simulink model "TIApplication"  (R2023b)
settings: Solver=FixedStepAuto  StartTime=0.0  StopTime=Inf  RelTol=1e-3  EnableMultiTasking=on
undefined symbols (not defined in the file): CountPerVolt, CurrentControl_I, CurrentControl_P, CurrentSensor_Bias, CurrentSensor_Gain, Down, FastSim_ElecTs, GPTRIP1SEL, GPTRIP2SEL, inverterBusVoltage, InverterCurrent_Max, InverterDCLink_Voltage, K, Ld, Lq, M, p, psim, pwmCounterMax, PWMMod_Period, PWMPercentAtZeroVolt, PWMPercentPerVolt, SpeedControl_I, SpeedControl_P, TI_ADCMax, TI_ADCMin, TI_ADCResolution, Tmax, TransducerVoltAtZeroAmpere, TransduceVoltPerAmpere, Ts, TZ1, TZ2, Up, ZeroVoltCount
libraries: mcbcontrolslib x9, c2802xlib x7, simulink x3, mcbpositiondecoderlib x3, slpidlib x3, idelinklib_common x2, c280xlib x2, mcbhdlpositiondecoderlib x2, eePmsmCurrentController x1, eeTransforms x1, eePwmGeneratorTwoLevel x1, eeLuenbergerObserver x1
(part 2 of 2)

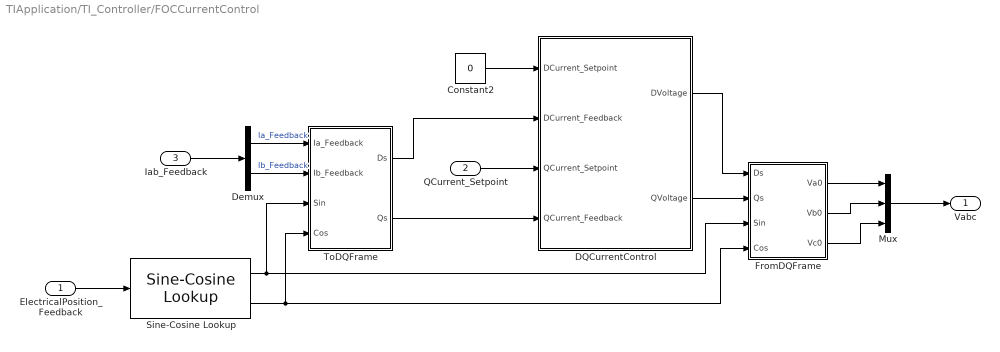
== system TIApplication/TI_Controller/FOCCurrentControl ==
  ElectricalPosition_Feedback : Inport
  QCurrent_Setpoint : Inport  Port=2
  Iab_Feedback : Inport  Port=3
  Constant2 : Constant  Value=0  OutDataTypeStr=Inherit: Inherit via back propagation  SampleTime=-1
  DQCurrentControl : Subsystem
  Demux : Demux  Outputs=2
  FromDQFrame : Subsystem
  Mux : Mux  Inputs=3
  Sine-Cosine Lookup : mcbcontrolslib/Sine-Cosine Lookup  AngleInput=Radians  N_points=1024
      settings: LibrarySourceBlock=mcblib/Controls/Math Transforms/Sine-Cosine Lookup
  ToDQFrame : Subsystem
  Vabc : Outport
  wires:
  Sine-Cosine Lookup/2 -> FromDQFrame/4(Cos), ToDQFrame/4(Cos)
  QCurrent_Setpoint/1 -> DQCurrentControl/3(QCurrent_Setpoint)
  Iab_Feedback/1 -> Demux/1
  Sine-Cosine Lookup/1 -> FromDQFrame/3(Sin), ToDQFrame/3(Sin)
  Constant2/1 -> DQCurrentControl/1(DCurrent_Setpoint)
  Mux/1 -> Vabc/1
  ElectricalPosition_Feedback/1 -> Sine-Cosine Lookup/1
  Demux/1 -> ToDQFrame/1(Ia_Feedback)  "Ia_Feedback"
  Demux/2 -> ToDQFrame/2(Ib_Feedback)  "Ib_Feedback"
  ToDQFrame/1(Ds) -> DQCurrentControl/2(DCurrent_Feedback)
  ToDQFrame/2(Qs) -> DQCurrentControl/4(QCurrent_Feedback)
  DQCurrentControl/1(DVoltage) -> FromDQFrame/1(Ds)
  DQCurrentControl/2(QVoltage) -> FromDQFrame/2(Qs)
  FromDQFrame/1(Va0) -> Mux/1
  FromDQFrame/2(Vb0) -> Mux/2
  FromDQFrame/3(Vc0) -> Mux/3

== system TIApplication/TI_Controller/PUToPWMPercent ==
  Vabc : Inport
  Add : Sum
  Constant : Constant  Value=PWMPercentPerVolt  OutDataTypeStr=Inherit: Inherit via back propagation  SampleTime=-1
  Constant2 : Constant  Value=PWMPercentAtZeroVolt  OutDataTypeStr=Inherit: Inherit via back propagation  SampleTime=-1
  Data Type Conversion : DataTypeConversion  OutDataTypeStr=uint16  SaturateOnIntegerOverflow=off  RndMeth=Floor
  Product : Product  OutDataTypeStr=Inherit: Inherit via back propagation
  Saturation : Saturate  UpperLimit=100  LowerLimit=0
  DutyCyclePercent : Outport
  wires:
  Vabc/1 -> Product/1
  Add/1 -> Saturation/1
  Constant/1 -> Product/2
  Product/1 -> Add/1
  Constant2/1 -> Add/2
  Saturation/1 -> Data Type Conversion/1
  Data Type Conversion/1 -> DutyCyclePercent/1

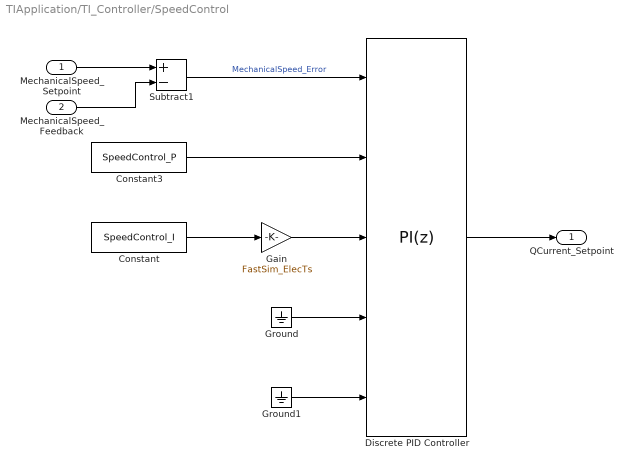
== system TIApplication/TI_Controller/SpeedControl ==
  MechanicalSpeed_Setpoint : Inport
  MechanicalSpeed_Feedback : Inport  Port=2
  Constant : Constant  Value=SpeedControl_I  OutDataTypeStr=Inherit: Inherit via back propagation  SampleTime=-1
  Constant3 : Constant  Value=SpeedControl_P  OutDataTypeStr=Inherit: Inherit via back propagation  SampleTime=-1
  Discrete PID Controller : slpidlib/PID Controller  Controller=PI  Form=Parallel  TimeDomain=Discrete-time  UseExternalTs=off  SampleTime=-1  IntegratorMethod=Forward Euler  FilterMethod=Forward Euler  ControllerParametersSource=external  P=1  I=1  UseKiTs=on  D=0  N=100  UseFilter=on  TunerSelectOption=Transfer Function Based (PID Tuner App)  InitialConditionSource=external  InitialConditionForIntegrator=0  InitialConditionForFilter=0  DifferentiatorICPrevScaledInput=0  ExternalReset=level  TrackingMode=off  Kt=1  LimitOutput=on  SatLimitsSource=internal  UpperSaturationLimit=InverterCurrent_Max  LowerSaturationLimit=-InverterCurrent_Max  LinearizeAsGain=on  AntiWindupMode=none  Kb=1  LimitIntegrator=off  UpperIntegratorSaturationLimit=inf  LowerIntegratorSaturationLimit=-inf  RndMeth=Simplest  POutMin=[]  POutMax=[]  IOutMin=[]  IOutMax=[]  DOutMin=[]  DOutMax=[]  NOutMin=[]  NOutMax=[]  SumOutMin=[]  SumOutMax=[]  SaturationOutMin=[]  SaturationOutMax=[]  PParamMin=[]  PParamMax=[]  IParamMin=[]  IParamMax=[]  DParamMin=[]  DParamMax=[]  NParamMin=[]  NParamMax=[]  KbParamMin=[]  KbParamMax=[]  KtParamMin=[]  KtParamMax=[]  KbOutMin=[]  KbOutMax=[]  KtOutMin=[]  KtOutMax=[]  IntegratorOutMin=[]  IntegratorOutMax=[]  FilterOutMin=[]  FilterOutMax=[]  SumI1OutMin=[]  SumI1OutMax=[]  SumI2OutMin=[]  SumI2OutMax=[]  SumI3OutMin=[]  SumI3OutMax=[]  SumI4OutMin=[]  SumI4OutMax=[]  SumDOutMin=[]  SumDOutMax=[]  DifferentiatorOutMin=[]  DifferentiatorOutMax=[]  FilterDiffOutCoefMin=[]  FilterDiffOutCoefMax=[]  ReciprocalOutMin=[]  ReciprocalOutMax=[]  SumDenOutMin=[]  SumDenOutMax=[]  SumNumOutMin=[]  SumNumOutMax=[]  DivideOutMin=[]  DivideOutMax=[]  UdiffTsProdOutMin=[]  UdiffTsProdOutMax=[]  NTsProdOutMin=[]  NTsProdOutMax=[]  UintegralTsProdOutMin=[]  UintegralTsProdOutMax=[]  UngainTsProdOutMin=[]  UngainTsProdOutMax=[]  ClampingZeroOutDataTypeStr=Inherit: Inherit via back propagation  ClampingZeroOutMin=[]  ClampingZeroOutMax=[]  FilterDenConstantOutDataTypeStr=Inherit: Inherit via back propagation  FilterDenConstantOutMin=[]  FilterDenConstantOutMax=[]  PCopyOutDataTypeStr=Inherit: Inherit via back propagation  PCopyOutMin=[]  PCopyOutMax=[]  NCopyOutDataTypeStr=Inherit: Inherit via back propagation  NCopyOutMin=[]  NCopyOutMax=[]  IntegratorContinuousStateAttributes=''  IntegratorStateMustResolveToSignalObject=off  IntegratorRTWStateStorageClass=Auto  FilterContinuousStateAttributes=''  FilterStateMustResolveToSignalObject=off  FilterRTWStateStorageClass=Auto  ParallelPVariant=ExternalParameters  IdealPVariant=Disabled  IVariant=ExternalParameters  DVariant=Disabled  IntegratorVariant=Discrete  SatVariant=Enabled  AWVariant=Passthrough  PCopyVariant=Disabled  TRVariant=Disabled  FdbkBlocksVariant=Forward  IdealPFdbkVariant=Disabled  SatFdbkVariant=Disabled  DerivativeFilterVariant=Disabled  NVariant=Disabled  NCopyVariant=Disabled_SignalSpec  FilterICVariant=Disabled  IntegratorICVariant=ExternalICs  ExternalResetVariant=ExternalReset  TRSumVariant=Passthrough  SumFdbkVariant=Disabled  SumVariant=Sum_PI  TsampFilterVariant=InternalTs  TsampNgainVariant=Passthrough  TsampIntegralVariant=Disabled_SignalSpec  ExternalSaturationOutDataTypeStr=Inherit: Same as second input
      settings: LibrarySourceBlock=simulink/Discrete/Discrete PID Controller
  Gain : Gain  Gain=FastSim_ElecTs
  Ground : Ground
  Ground1 : Ground
  Subtract1 : Sum  Inputs=+-
  QCurrent_Setpoint : Outport
  wires:
  Constant/1 -> Gain/1
  MechanicalSpeed_Feedback/1 -> Subtract1/2
  Ground/1 -> Discrete PID Controller/4
  Subtract1/1 -> Discrete PID Controller/1  "MechanicalSpeed_Error"
  Constant3/1 -> Discrete PID Controller/2
  Gain/1 -> Discrete PID Controller/3
  Discrete PID Controller/1 -> QCurrent_Setpoint/1
  MechanicalSpeed_Setpoint/1 -> Subtract1/1
  Ground1/1 -> Discrete PID Controller/5

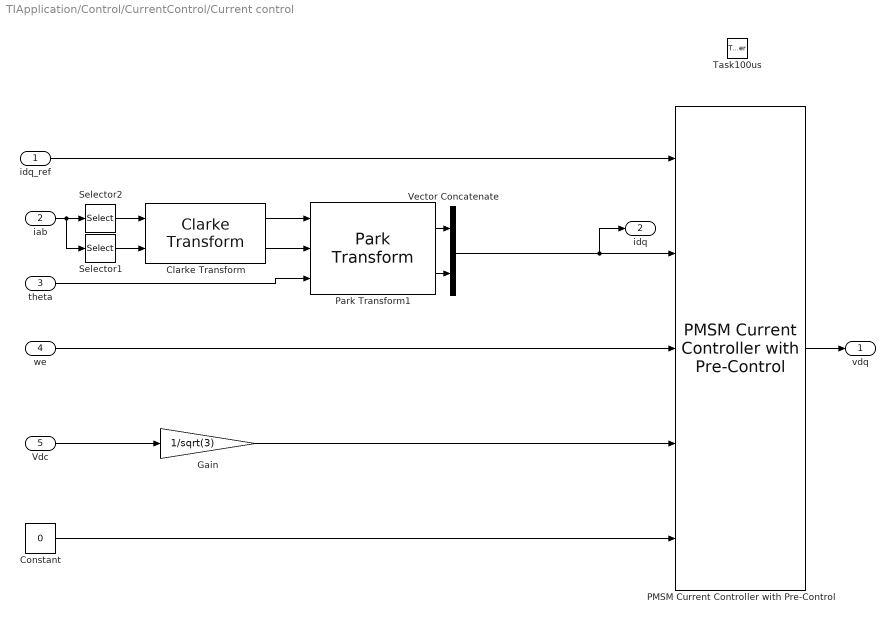
== system TIApplication/Control/CurrentControl/Current control ==
  idq_ref : Inport
  iab : Inport  Port=2
  theta : Inport  Port=3
  we : Inport  Port=4
  Vdc : Inport  Port=5
  Task100us : TriggerPort  TriggerType=function-call  VariantControl=Variant  PortDimensions=1
  Clarke Transform : mcbcontrolslib/Clarke Transform  VariantControl=Variant2  PhaseInput=Two inputs  EnPowerInv=off
      settings: LibrarySourceBlock=mcblib/Controls/Math Transforms/Clarke Transform
  Constant : Constant  Value=0  SampleTime=-1
  Gain : Gain  Gain=1/sqrt(3)
  PMSM Current Controller with Pre-Control : eePmsmCurrentController/PMSM Current Controller with Pre-Control  Kp_id=Kp_id  Ki_id=Ki_id  Kaw_id=1  Kp_iq=Kp_iq  Ki_iq=Ki_iq  Kaw_iq=1  Ts=-1  Tsd=Tsi  AxisPrio=D-Q equivalence  ActZC=on  ActFF=on  idVect=[-200, 0, 200]  iqVect=[-200, 0, 200]  LdMatrix=Ld * ones(3, 3)  LqMatrix=Lq * ones(3, 3)  psimMatrix=psim * ones(3, 3)
  Park Transform1 : mcbcontrolslib/Park Transform  PhaseInput=Two inputs  AxisAlignment=D-axis  ThetaInput=Electrical position  AngleInput=Radians  N_points=1024
      settings: LibrarySourceBlock=mcblib/Controls/Math Transforms/Park Transform
  Selector1 : Selector  InputPortWidth=2  IndexOptions=Index vector (dialog)  Indices=2  OutputSizes=1
  Selector2 : Selector  InputPortWidth=2  IndexOptions=Index vector (dialog)  Indices=1  OutputSizes=1
  Vector Concatenate : Concatenate
  vdq : Outport  VectorParamsAs1DForOutWhenUnconnected=off
  idq : Outport  Port=2  VectorParamsAs1DForOutWhenUnconnected=off
  wires:
  Vdc/1 -> Gain/1
  we/1 -> PMSM Current Controller with Pre-Control/3
  PMSM Current Controller with Pre-Control/1 -> vdq/1
  idq_ref/1 -> PMSM Current Controller with Pre-Control/1
  Constant/1 -> PMSM Current Controller with Pre-Control/5
  Vector Concatenate/1 -> idq/1, PMSM Current Controller with Pre-Control/2
  Gain/1 -> PMSM Current Controller with Pre-Control/4
  Clarke Transform/1 -> Park Transform1/1
  Clarke Transform/2 -> Park Transform1/2
  Park Transform1/2 -> Vector Concatenate/2
  Park Transform1/1 -> Vector Concatenate/1
  Selector2/1 -> Clarke Transform/1
  Selector1/1 -> Clarke Transform/2
  iab/1 -> Selector1/1, Selector2/1
  theta/1 -> Park Transform1/3

== system TIApplication/Control/Measurements/CurrentSensor_Inverse ==
  In1 : Inport
  InverseGain : Gain  Gain=1/CurrentSensor_Gain
  NegativeBias : Bias  Bias=-CurrentSensor_Bias  SaturateOnIntegerOverflow=off
  Out1 : Outport
  wires:
  In1/1 -> NegativeBias/1
  InverseGain/1 -> Out1/1
  NegativeBias/1 -> InverseGain/1

== system TIApplication/Control/Measurements/Vdc Filter ==
  In : Inport
  Discrete Transfer Fcn : DiscreteTransferFcn  Numerator=num  Denominator=den
  Out : Outport  VectorParamsAs1DForOutWhenUnconnected=off
  wires:
  Discrete Transfer Fcn/1 -> Out/1
  In/1 -> Discrete Transfer Fcn/1

== system TIApplication/TI_Controller/FOCCurrentControl/DQCurrentControl ==
  DCurrent_Setpoint : Inport
  DCurrent_Feedback : Inport  Port=2
  QCurrent_Setpoint : Inport  Port=3
  QCurrent_Feedback : Inport  Port=4
  DCurrentControl : Subsystem
  DQ Limiter : mcbcontrolslib/DQ Limiter  satMethodInputType=Specify via dialog  satMethodSelected=D-Q equivalence  satLimitInputType=Specify via dialog  Vmax=inverterBusVoltage/sqrt(3)
      settings: LibrarySourceBlock=mcbhdllib/Controls/Control Reference/DQ Limiter
  QCurrentControl : Subsystem
  Terminator : Terminator
  DVoltage : Outport
  QVoltage : Outport  Port=2
  wires:
  DCurrent_Feedback/1 -> DCurrentControl/2(Current_Feedback)
  QCurrent_Feedback/1 -> QCurrentControl/2(Current_Feedback)
  QCurrent_Setpoint/1 -> QCurrentControl/1(Current_Setpoint)
  DCurrentControl/1(Voltage) -> DQ Limiter/1
  QCurrentControl/1(Voltage) -> DQ Limiter/2
  DCurrent_Setpoint/1 -> DCurrentControl/1(Current_Setpoint)
  DQ Limiter/1 -> DVoltage/1
  DQ Limiter/2 -> QVoltage/1
  DQ Limiter/3 -> Terminator/1

== system TIApplication/TI_Controller/FOCCurrentControl/FromDQFrame ==
  Ds : Inport
  Qs : Inport  Port=2
  Sin : Inport  Port=3
  Cos : Inport  Port=4
  Inverse Park Transform : mcbcontrolslib/Inverse Park Transform  PhaseInput=Two inputs  AxisAlignment=D-axis  ThetaInput=Sine and Cosine electrical position  AngleInput=Per-unit  N_points=1024
      settings: LibrarySourceBlock=mcbhdllib/Controls/Math Transforms/Inverse Park Transform
  PWM Reference Generator : mcbcontrolslib/PWM Reference Generator  inSignal=Valphabeta  modType=SPWM: sinusoidal PWM
      settings: LibrarySourceBlock=mcblib/Controls/Math Transforms/PWM Reference Generator
  Va0 : Outport
  Vb0 : Outport  Port=2
  Vc0 : Outport  Port=3
  wires:
  Inverse Park Transform/1 -> PWM Reference Generator/1
  Qs/1 -> Inverse Park Transform/2
  Inverse Park Transform/2 -> PWM Reference Generator/2
  PWM Reference Generator/3 -> Vc0/1
  PWM Reference Generator/2 -> Vb0/1
  PWM Reference Generator/1 -> Va0/1
  Cos/1 -> Inverse Park Transform/4
  Ds/1 -> Inverse Park Transform/1
  Sin/1 -> Inverse Park Transform/3

== system TIApplication/TI_Controller/FOCCurrentControl/ToDQFrame ==
  Ia_Feedback : Inport
  Ib_Feedback : Inport  Port=2
  Sin : Inport  Port=3
  Cos : Inport  Port=4
  Clarke Transform : mcbcontrolslib/Clarke Transform  VariantControl=Variant2  PhaseInput=Two inputs  EnPowerInv=off
      settings: LibrarySourceBlock=mcbhdllib/Controls/Math Transforms/Clarke Transform
  Park Transform : mcbcontrolslib/Park Transform  PhaseInput=Two inputs  AxisAlignment=D-axis  ThetaInput=Sine and Cosine electrical position  AngleInput=Per-unit  N_points=1024
      settings: LibrarySourceBlock=mcbhdllib/Controls/Math Transforms/Park Transform
  Ds : Outport
  Qs : Outport  Port=2
  wires:
  Clarke Transform/1 -> Park Transform/1
  Ib_Feedback/1 -> Clarke Transform/2
  Clarke Transform/2 -> Park Transform/2
  Park Transform/2 -> Qs/1
  Ia_Feedback/1 -> Clarke Transform/1
  Sin/1 -> Park Transform/3
  Park Transform/1 -> Ds/1
  Cos/1 -> Park Transform/4

== system TIApplication/TI_Controller/FOCCurrentControl/DQCurrentControl/DCurrentControl ==
  Current_Setpoint : Inport
  Current_Feedback : Inport  Port=2
  Constant2 : Constant  Value=CurrentControl_P  SampleTime=-1
  Constant3 : Constant  Value=CurrentControl_I  SampleTime=-1
  Constant4 : Constant  Value=0  OutDataTypeStr=Inherit: Inherit via back propagation  SampleTime=-1
  Discrete PID Controller : slpidlib/PID Controller  Controller=PI  Form=Parallel  TimeDomain=Discrete-time  UseExternalTs=off  SampleTime=-1  IntegratorMethod=Forward Euler  FilterMethod=Forward Euler  ControllerParametersSource=external  P=1  I=1  UseKiTs=on  D=0  N=100  UseFilter=on  TunerSelectOption=Transfer Function Based (PID Tuner App)  InitialConditionSource=external  InitialConditionForIntegrator=0  InitialConditionForFilter=0  DifferentiatorICPrevScaledInput=0  ExternalReset=level  TrackingMode=off  Kt=1  LimitOutput=on  SatLimitsSource=internal  UpperSaturationLimit=InverterDCLink_Voltage/sqrt(3)  LowerSaturationLimit=-InverterDCLink_Voltage/sqrt(3)  LinearizeAsGain=off  AntiWindupMode=clamping  Kb=1  LimitIntegrator=off  UpperIntegratorSaturationLimit=inf  LowerIntegratorSaturationLimit=-inf  RndMeth=Simplest  POutMin=[]  POutMax=[]  IOutMin=[]  IOutMax=[]  DOutMin=[]  DOutMax=[]  NOutMin=[]  NOutMax=[]  SumOutMin=[]  SumOutMax=[]  SaturationOutDataTypeStr=Inherit: Inherit via back propagation  SaturationOutMin=[]  SaturationOutMax=[]  PParamMin=[]  PParamMax=[]  IParamMin=[]  IParamMax=[]  DParamMin=[]  DParamMax=[]  NParamMin=[]  NParamMax=[]  KbParamMin=[]  KbParamMax=[]  KtParamMin=[]  KtParamMax=[]  KbOutMin=[]  KbOutMax=[]  KtOutMin=[]  KtOutMax=[]  IntegratorOutMin=[]  IntegratorOutMax=[]  FilterOutMin=[]  FilterOutMax=[]  SumI1OutMin=[]  SumI1OutMax=[]  SumI2OutMin=[]  SumI2OutMax=[]  SumI3OutMin=[]  SumI3OutMax=[]  SumI4OutMin=[]  SumI4OutMax=[]  SumDOutMin=[]  SumDOutMax=[]  DifferentiatorOutMin=[]  DifferentiatorOutMax=[]  FilterDiffOutCoefMin=[]  FilterDiffOutCoefMax=[]  ReciprocalOutMin=[]  ReciprocalOutMax=[]  SumDenOutMin=[]  SumDenOutMax=[]  SumNumOutMin=[]  SumNumOutMax=[]  DivideOutMin=[]  DivideOutMax=[]  UdiffTsProdOutMin=[]  UdiffTsProdOutMax=[]  NTsProdOutMin=[]  NTsProdOutMax=[]  UintegralTsProdOutMin=[]  UintegralTsProdOutMax=[]  UngainTsProdOutMin=[]  UngainTsProdOutMax=[]  ClampingZeroOutDataTypeStr=Inherit: Inherit via back propagation  ClampingZeroOutMin=[]  ClampingZeroOutMax=[]  FilterDenConstantOutDataTypeStr=Inherit: Inherit via back propagation  FilterDenConstantOutMin=[]  FilterDenConstantOutMax=[]  PCopyOutDataTypeStr=Inherit: Inherit via back propagation  PCopyOutMin=[]  PCopyOutMax=[]  NCopyOutDataTypeStr=Inherit: Inherit via back propagation  NCopyOutMin=[]  NCopyOutMax=[]  IntegratorContinuousStateAttributes=''  IntegratorStateMustResolveToSignalObject=off  IntegratorRTWStateStorageClass=Auto  FilterContinuousStateAttributes=''  FilterStateMustResolveToSignalObject=off  FilterRTWStateStorageClass=Auto  ParallelPVariant=ExternalParameters  IdealPVariant=Disabled  IVariant=ExternalParameters  DVariant=Disabled  IntegratorVariant=Discrete  SatVariant=Enabled  AWVariant=DiscClampingParallel  PCopyVariant=Disabled  TRVariant=Disabled  FdbkBlocksVariant=Forward  IdealPFdbkVariant=Disabled  SatFdbkVariant=Disabled  DerivativeFilterVariant=Disabled  NVariant=Disabled  NCopyVariant=Disabled_SignalSpec  FilterICVariant=Disabled  IntegratorICVariant=ExternalICs  ExternalResetVariant=ExternalReset  TRSumVariant=Passthrough  SumFdbkVariant=Disabled  SumVariant=Sum_PI  TsampFilterVariant=InternalTs  TsampNgainVariant=Passthrough  TsampIntegralVariant=Disabled_SignalSpec  ExternalSaturationOutDataTypeStr=Inherit: Same as second input
      settings: LibrarySourceBlock=simulink/Discrete/Discrete PID Controller
  Error : Sum  Inputs=+-
  Gain1 : Gain  Gain=FastSim_ElecTs
  Ground : Ground
  Voltage : Outport
  wires:
  Constant2/1 -> Discrete PID Controller/2
  Constant4/1 -> Discrete PID Controller/5
  Discrete PID Controller/1 -> Voltage/1
  Error/1 -> Discrete PID Controller/1  "Current_Error"
  Current_Setpoint/1 -> Error/1
  Constant3/1 -> Gain1/1
  Gain1/1 -> Discrete PID Controller/3
  Ground/1 -> Discrete PID Controller/4
  Current_Feedback/1 -> Error/2

== system TIApplication/TI_Controller/FOCCurrentControl/DQCurrentControl/QCurrentControl ==
  Current_Setpoint : Inport
  Current_Feedback : Inport  Port=2
  Constant2 : Constant  Value=CurrentControl_P  OutDataTypeStr=Inherit: Inherit via back propagation
  Constant3 : Constant  Value=CurrentControl_I  OutDataTypeStr=Inherit: Inherit via back propagation
  Constant4 : Constant  Value=0  OutDataTypeStr=Inherit: Inherit via back propagation
  Discrete PID Controller : slpidlib/PID Controller  Controller=PI  Form=Parallel  TimeDomain=Discrete-time  UseExternalTs=off  SampleTime=-1  IntegratorMethod=Forward Euler  FilterMethod=Forward Euler  ControllerParametersSource=external  P=1  I=1  UseKiTs=on  D=0  N=100  UseFilter=on  TunerSelectOption=Transfer Function Based (PID Tuner App)  InitialConditionSource=external  InitialConditionForIntegrator=0  InitialConditionForFilter=0  DifferentiatorICPrevScaledInput=0  ExternalReset=level  TrackingMode=off  Kt=1  LimitOutput=on  SatLimitsSource=internal  UpperSaturationLimit=InverterDCLink_Voltage/sqrt(3)  LowerSaturationLimit=-InverterDCLink_Voltage/sqrt(3)  LinearizeAsGain=off  AntiWindupMode=clamping  Kb=1  LimitIntegrator=off  UpperIntegratorSaturationLimit=inf  LowerIntegratorSaturationLimit=-inf  POutMin=[]  POutMax=[]  IOutMin=[]  IOutMax=[]  DOutMin=[]  DOutMax=[]  NOutMin=[]  NOutMax=[]  SumOutMin=[]  SumOutMax=[]  SaturationOutDataTypeStr=Inherit: Inherit via back propagation  SaturationOutMin=[]  SaturationOutMax=[]  PParamMin=[]  PParamMax=[]  IParamMin=[]  IParamMax=[]  DParamMin=[]  DParamMax=[]  NParamMin=[]  NParamMax=[]  KbParamMin=[]  KbParamMax=[]  KtParamMin=[]  KtParamMax=[]  KbOutMin=[]  KbOutMax=[]  KtOutMin=[]  KtOutMax=[]  IntegratorOutMin=[]  IntegratorOutMax=[]  FilterOutMin=[]  FilterOutMax=[]  SumI1OutMin=[]  SumI1OutMax=[]  SumI2OutMin=[]  SumI2OutMax=[]  SumI3OutMin=[]  SumI3OutMax=[]  SumI4OutMin=[]  SumI4OutMax=[]  SumDOutMin=[]  SumDOutMax=[]  DifferentiatorOutMin=[]  DifferentiatorOutMax=[]  FilterDiffOutCoefMin=[]  FilterDiffOutCoefMax=[]  ReciprocalOutMin=[]  ReciprocalOutMax=[]  SumDenOutMin=[]  SumDenOutMax=[]  SumNumOutMin=[]  SumNumOutMax=[]  DivideOutMin=[]  DivideOutMax=[]  UdiffTsProdOutMin=[]  UdiffTsProdOutMax=[]  NTsProdOutMin=[]  NTsProdOutMax=[]  UintegralTsProdOutMin=[]  UintegralTsProdOutMax=[]  UngainTsProdOutMin=[]  UngainTsProdOutMax=[]  ClampingZeroOutDataTypeStr=Inherit: Inherit via back propagation  ClampingZeroOutMin=[]  ClampingZeroOutMax=[]  FilterDenConstantOutDataTypeStr=Inherit: Inherit via back propagation  FilterDenConstantOutMin=[]  FilterDenConstantOutMax=[]  PCopyOutDataTypeStr=Inherit: Inherit via back propagation  PCopyOutMin=[]  PCopyOutMax=[]  NCopyOutDataTypeStr=Inherit: Inherit via back propagation  NCopyOutMin=[]  NCopyOutMax=[]  IntegratorContinuousStateAttributes=''  IntegratorStateMustResolveToSignalObject=off  IntegratorRTWStateStorageClass=Auto  FilterContinuousStateAttributes=''  FilterStateMustResolveToSignalObject=off  FilterRTWStateStorageClass=Auto  ParallelPVariant=ExternalParameters  IdealPVariant=Disabled  IVariant=ExternalParameters  DVariant=Disabled  IntegratorVariant=Discrete  SatVariant=Enabled  AWVariant=DiscClampingParallel  PCopyVariant=Disabled  TRVariant=Disabled  FdbkBlocksVariant=Forward  IdealPFdbkVariant=Disabled  SatFdbkVariant=Disabled  DerivativeFilterVariant=Disabled  NVariant=Disabled  NCopyVariant=Disabled_SignalSpec  FilterICVariant=Disabled  IntegratorICVariant=ExternalICs  ExternalResetVariant=ExternalReset  TRSumVariant=Passthrough  SumFdbkVariant=Disabled  SumVariant=Sum_PI  TsampFilterVariant=InternalTs  TsampNgainVariant=Passthrough  TsampIntegralVariant=Disabled_SignalSpec  ExternalSaturationOutDataTypeStr=Inherit: Same as second input
      settings: LibrarySourceBlock=simulink/Discrete/Discrete PID Controller
  Error : Sum  Inputs=+-
  Gain : Gain  Gain=FastSim_ElecTs
  Ground : Ground
  Voltage : Outport
  wires:
  Current_Feedback/1 -> Error/2
  Ground/1 -> Discrete PID Controller/4
  Gain/1 -> Discrete PID Controller/3
  Constant3/1 -> Gain/1
  Current_Setpoint/1 -> Error/1
  Error/1 -> Discrete PID Controller/1  "Current_Error"
  Discrete PID Controller/1 -> Voltage/1
  Constant4/1 -> Discrete PID Controller/5
  Constant2/1 -> Discrete PID Controller/2
